simulink model "uas_main_ros2"  (R2026a)
settings: Solver=FixedStepAuto  StopTime=Inf  FixedStep=sample_time
model workspace: external: MAT-File (data not in the file)
values from neighbouring files (symbols this model uses):
  arm_length = 0.17    [uas_parameters.m]
  axes_msg = zeros(1, 124)    [uas_parameters.m]
  button_msg = zeros(1, 124)    [uas_parameters.m]
  drag_coefficient = 0.47    [uas_parameters.m]
  g = 9.81    [PosControllerSystem.m]    (also in uas_parameters.m = 9.80665)
  inertia_xx = 0.007    [uas_parameters.m]
  inertia_yy = 0.007    [uas_parameters.m]
  inertia_zz = 0.012    [uas_parameters.m]
  mass_drone = 0.04    [uas_parameters.m]
  mass_total = 0.04    [PosControllerSystem.m]    (also in uas_parameters.m)
  max_rot_velocity = 838    [uas_parameters.m]
  mix_matrix = inv(motor_constant * allocation_matrix)    [uas_parameters.m]
  moment_constant = 0.016    [uas_parameters.m]
  motor_constant = 8.54858e-06    [uas_parameters.m]
  N = size(waypoints, 1)    [quintic_interp.m]
  reference_area = pi * 75e-3^2    (= 0.0176714586764)    [uas_parameters.m]
  rotor_offset_top = 0.01    [uas_parameters.m]
  route = [0 0 1 ; 9 0 1 ; 9 9 1]    [uas_parameters.m]
  sample_time = 4e-2    (= 0.04)    [uas_parameters.m]
  x0 = 36    [uas_parameters.m]
  y0 = 80    [uas_parameters.m]
  z0 = 1    [uas_parameters.m]
undefined symbols (not defined in the file or in its folder): axes, axes_SL_Info, buttons, buttons_SL_Info, poly_traj, quat2rotm, X, Y, Z
libraries: nesl_utility x32, sm_lib x25, ros2lib x16, dspfdesign x3, simulink x2, sharedtransform x2, sim3dlib x1, uavsim3dlib x1, vrlib x1
(part 1 of 3)
settings Model: Creator=david  LastModifiedBy=mello
settings OptimizationCC: PassReuseOutputArgsThreshold=0.0
settings DebuggingCC: UnderSpecifiedDimensionMsg=warning
settings HardwareCC: ProdHWDeviceType=Generic->Unspecified (assume 32-bit Generic)  UseEmbeddedCoderFeatures=off
settings SFSimCC: SimTargetLang=C++
settings RTWCC: SystemTargetFile=ert.tlc  HardwareBoard=Robot Operating System (ROS)  TLCOptions="-aInlineSetEventsForThisBaseRateFcn=TLC_FALSE -aSuppressMultiTaskScheduler=TLC_FALSE  -aRateBasedStepFcn=0"  Toolchain=Catkin  TargetLang=C++  Description=Embedded Coder
settings ERTTargetCC: RootIOFormat=Structure reference  DynamicArrayContainerType=coder::array  ERTCustomFileBanners=off  CodeInterfacePackaging=C++ class  SupportContinuousTime=on  SupportNonInlinedSFcns=on  ModelStepFunctionPrototypeControlCompliant=off
settings SimscapeCC: SimscapeNominalValues="[{\"value\":\"1\",\"unit\":\"A\"},{\"value\":\"1\",\"unit\":\"bar\"},{\"value\":\"1\",\"unit\":\"cm^2\"},{\"value\":\"1\",\"unit\":\"cm^3/s\"},{\"value\":\"1\",\"unit\":\"kJ/kg\"},{\"value\":\"1\",\"unit\":\"kW\"},{\"value\":\"1\",\"unit\":\"l\"},{\"value\":\"1\",\"unit\":\"N\"},{\"value\":\"1\",\"unit\":\"N*m\"},{\"value\":\"1\",\"unit\":\"V\"}]"  SimscapeLogSimulationStatistics=on
settings ExplorerConfigSet: InternalSimMechanicsExplorerSettings="<ExplorerConfiguration><canonicalview>default</canonicalview><AnimationSetting><BasePlaybackSpeed>1.0</BasePlaybackSpeed><PlaybackSpeedFactor>1.0</PlaybackSpeedFactor></AnimationSetting><TilePanel><TileInfo><Tiles Columns=\"1\" Count=\"1\" Rows=\"1\"><Column Weight=\"1\"/><Row Weight=\"1\"/><Tile Height=\"1\" Width=\"1\" X=\"0\" Y=\"0\"/></Tiles></TileInfo><SceneInfo><SceneViewer><BGColor><R>0.400000005960464478</R><G>0.400000005960464478</G><B>0.400000005960464478</B></BGColor><Camera><DoPerspective>off</DoPerspective><Position><X>7.41918867546502359</X><Y>0.562842449888731333</Y><Z>8.36768126399918444</Z></Position><Center><X>4.24878770726833288</X><Y>4.27540210027623324</Y><Z>0.996100590645515815</Z></Center><Up><X>-0.578313069199200891</X><Y>0.601173295476169489</Y><Z>0.551493121262380703</Z></Up><ViewLimDist>1</ViewLimDist><YLim>5.48746925830841104</YLim><XLim>8.41878250057976274</XLim></Camera></SceneViewer></SceneInfo></TilePanel><MechEditorPanel><Cameras/><GfxPanelCameraMap/><VideoCreator><PlaybackSpeedRatio>1.0</PlaybackSpeedRatio><FrameRate>30</FrameRate><VideoFormat>Motion JPEG AVI</VideoFormat><FrameSize>auto</FrameSize></VideoCreator></MechEditorPanel></ExplorerConfiguration>"

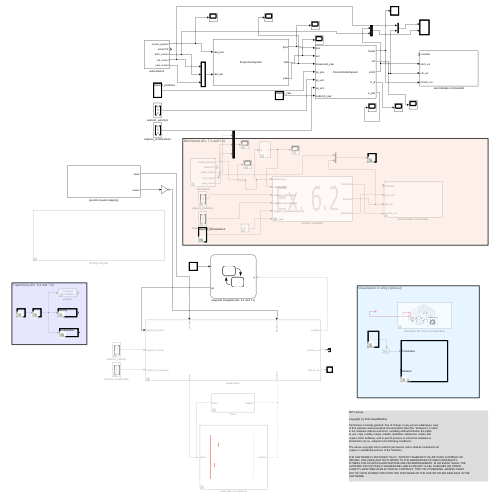
[thumbnail: Simulink's stored preview of the top-level diagram]
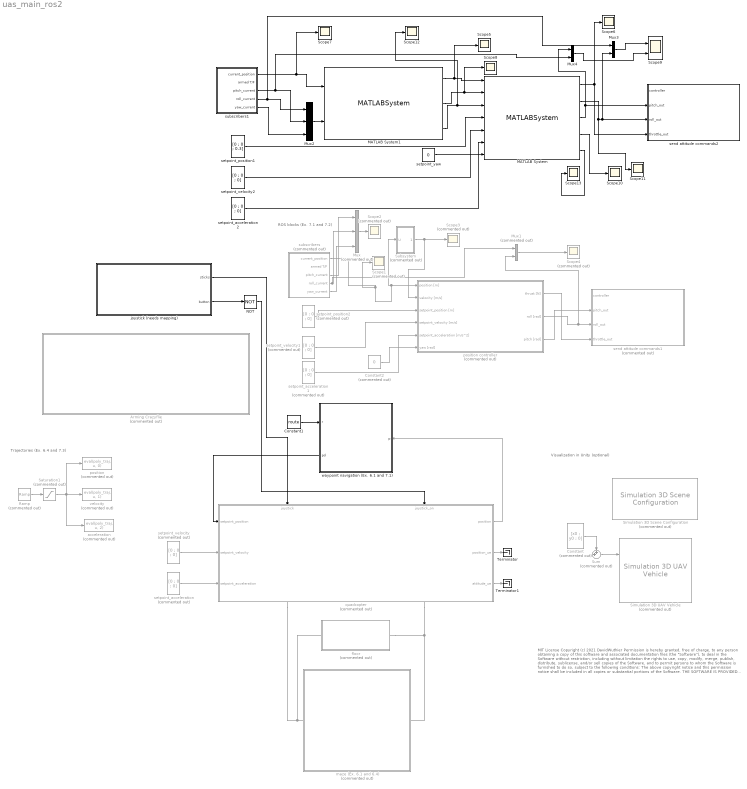
== system uas_main_ros2 ==
  note: MIT License
      |
      | Copyright (c) 2021 DavidWuthier
      |
      | Permission is hereby granted, free of charge, to any person obtaining a copy
      | of this software and associated documentation files (the "Software"), to deal
      | in the Software without restriction, including without limitation the rights
      | to use, copy, modify, merge, publish, distribute, sublicense, and/or sell
      | copies of the Software, and to permit persons to whom the Software is
      | furnished to do so, subject to the following conditions:
      |
      | The above copyright notice and this permission notice shall be included in all
      | copies or substantial portions of the Software.
      |
      | THE SOFTWARE IS PROVIDED "AS IS", WITHOUT WARRANTY OF ANY KIND, EXPRESS OR
      | IMPLIED, INCLUDING BUT NOT LIMITED TO THE WARRANTIES OF MERCHANTABILITY,
      | FITNESS FOR A PARTICULAR PURPOSE AND NONINFRINGEMENT. IN NO EVENT SHALL THE
      | AUTHORS OR COPYRIGHT HOLDERS BE LIABLE FOR ANY CLAIM, DAMAGES OR OTHER
      | LIABILITY, WHETHER IN AN ACTION OF CONTRACT, TORT OR OTHERWISE, ARISING FROM,
      | OUT OF OR IN CONNECTION WITH THE SOFTWARE OR THE USE OR OTHER DEALINGS IN THE
      | SOFTWARE.
  note: Visualization in Unity (optional)
  note: Trajectories (Ex. 6.4 and 7.3)
  note: ROS blocks (Ex. 7.1 and 7.2)
  Arming Crazyflie : Subsystem  Commented=on
  Constant : Constant  Commented=on  Value=[x0 ; y0 ; 0]  VectorParams1D=off
  Constant1 : Constant  Value=route
  Constant2 : Constant  Commented=on  Value=0
  MATLAB System : MATLABSystem  System=PosControllerSystem  SimulateUsing=Code generation
      mask Type: PosControllerSystem
  MATLAB System1 : MATLABSystem  System=PreprocessSystem  SimulateUsing=Interpreted execution
      mask Type: PreprocessSystem
  Mux : Mux  Commented=on  Inputs=3
  Mux1 : Mux  Commented=on  Inputs=2
  Mux2 : Mux  Inputs=3
  Mux3 : Mux  Inputs=2
  Mux4 : Mux  Inputs=2
  NOT : Logic  Operator=NOT  IconShape=distinctive  AllPortsSameDT=off  OutDataTypeStr=boolean
  Ramp : simulink/Sources/Ramp  Commented=on  slope=1  start=0  InitialOutput=0
  Saturation1 : Saturate  Commented=on  UpperLimit=knots(end)  LowerLimit=0
  Scope{1..4} (4 alike) : Scope  Commented=on
      Scope1 settings: ActiveDisplayYMinimum=-3.62331068311887  ActiveDisplayYMaximum=5.4527683046975284  DataLoggingVariableName=ScopeData2
      Scope2 settings: ActiveDisplayYMinimum=-3.9205477094873689  ActiveDisplayYMaximum=3.9221624092985992  DataLoggingVariableName=ScopeData8
      Scope3 settings: ActiveDisplayYMinimum=-0.704351972070756  ActiveDisplayYMaximum=1.1465122899088067
      Scope4 settings: ActiveDisplayYMinimum=-2.2453805222482135  ActiveDisplayYMaximum=0.97073912636413651  DataLoggingVariableName=ScopeData9
  Scope{5..8,10..13} (8 alike) : Scope
      Scope10 settings: ActiveDisplayYMinimum=-0.2913419984889255  ActiveDisplayYMaximum=0.16018686807512672  DataLoggingVariableName=ScopeData16
      Scope11 settings: ActiveDisplayYMinimum=-7.8906329945921971  ActiveDisplayYMaximum=8.2581334209704433  DataLoggingVariableName=ScopeData17
      Scope12 settings: ActiveDisplayYMinimum=-3.5797770650115455  ActiveDisplayYMaximum=6.1446597978088091  DataLoggingVariableName=ScopeData18
      Scope13 settings: ActiveDisplayYMinimum=-2.1801041636378873  ActiveDisplayYMaximum=1.2366941298563761  DataLoggingVariableName=ScopeData19
      Scope5 settings: ActiveDisplayYMinimum=-1.3039902181688128  ActiveDisplayYMaximum=1.1270222818311879  DataLoggingVariableName=ScopeData10
      Scope6 settings: ActiveDisplayYMinimum=-0.96457637394383644  ActiveDisplayYMaximum=1.4435775810644444  DataLoggingVariableName=ScopeData11
      Scope7 settings: ActiveDisplayYMinimum=-18.731354302133511  ActiveDisplayYMaximum=13.426335857782668  DataLoggingVariableName=ScopeData12
      Scope8 settings: ActiveDisplayYMinimum=-3.9205477094873689  ActiveDisplayYMaximum=3.9221624092985992  DataLoggingVariableName=ScopeData13
  Scope9 : Scope  NumInputPorts=2
      settings: ActiveDisplayYMinimum=-11.154686865264761  ActiveDisplayYMaximum=4.93616611048231  DataLoggingVariableName=ScopeData15
  Simulation 3D Scene Configuration : sim3dlib/Simulation 3D Scene Configuration  Priority=0  Commented=on  ProjectFormat=Default Scenes  SceneDesc=US city block  ProjectName=/usr/local/MATLAB/R2026a/toolbox/shared/sim3d_projects/automotive_project_linux/UE/LinuxNoEditor/VehicleSimulation.sh  ScenePath=/Game/Maps/USCityBlock  EnableOpenDRIVE=off  vehTagList={'Scene Origin';'SimulinkVehicle1'}  vehTag=SimulinkVehicle1  AttachedCameraRelativeTranslation=[0 0 0]  FreeCameraDefaultInitialTranslation=[-6, 0, 2]  AttachedCameraRelativeRotation=[0 0 0]  FreeCameraDefaultInitialRotation=[0, -15, 0]  ViewpointName=Custom  FreeCameraInitialTranslation=[0, 0, 0]  FreeCameraInitialRotation=[0, 0, 0]  OpVisEn=off  Ts=sample_time  EnableWindow=on  EnableRemoteAccess=off  SimulationMode=CoSimulation  SimulateUsing=Interpreted execution  EnableAnimationRecording=off  OverrideDefaultRecording=off  AnimationRecordingFileName=sim3dAnimation.mat  AnimationRecordingInterval=[0 inf]  EnableWeather=off  SunAzimuth=90  SunAltitude=40.0  EnableGeospatialSun=off  Latitude=0  Longitude=0  Date=2023-01-01  Time=10:30:00  GeoTimeZone=-5.0  SunDaylightSaving=off  wind=1  clouds=10  EnableVolumetricClouds=off  CloudCoverage=0  CloudAltitude=6  fog=0  rain=0  RaindropsEffect=off  SnowDensity=0  EnableGeospatial=off  TilesetSource=Earth terrain  UseTrueOrigin=off  OriginHeight=200  OriginLatitude=40.744652  OriginLongitude=-73.988864  MapStyle=Aerial  AdditionalAssetIDs=[]  UseAdvancedSunSky=off  SolarTime=11  TimeZone=-5  Day=21  Month=9  Year=2022  UseDaylightSavingTime=on  DSTStartDay=10  DSTStartMonth=3  DSTEndDay=3  DSTEndMonth=11  DSTSwitchHour=2  sensorTag=MainCamera1  sensorId=1  sensorName=MainCamera1  mountLoc=Origin  offsetFlag=off  tmountOffset=[0, 0, 0]  rmountOffset=[0, 0, 0]  HorizontalResolution=1280  VerticalResolution=720  HorizontalFOV=60  mountPoint=[0 0 0]  mountOrientation=[0 0 0]  aMode=4  ID=1  GeoTrigger=Inactive  ViewNameList={'Custom'}  ViewTranslationList={'[0 0 0]'}  ViewRotationList={'[0 0 0]'}
      settings: LibrarySourceBlock=uavsim3dlib/Simulation 3D Scene Configuration
  Simulation 3D UAV Vehicle : uavsim3dlib/Simulation 3D UAV Vehicle  Commented=on  Mesh=Quadrotor  MeshPath=/MathWorksUAVContent/UAVs/HexaRotorUAV/HexaRotor.HexaRotor  Color=Black  ActorName=SimulinkVehicle1  UseGlobalFrame=off  InitialTranslation=[x0 y0 z0]  InitialRotation=[0 0 0]  InitialTranslationGlobal=[0 0 0]  InitialGeoOrigin=[0 0 0]  InitialRotationGlobal=[0 0 0]  SampleTime=-1  ActorType=SimulinkVehicle  ID=1  aMode=4  ActorTag=SimulinkVehicle1
  Subsystem : Subsystem  Commented=on
  Sum : Sum  Commented=on  Inputs=++|
  Terminator : Terminator
  Terminator1 : Terminator
  acceleration : MATLABFcn  Commented=on  MATLABFcn=eval(poly_traj, u, 2)  OutputDimensions=[3 1]  Output1D=off
  floor : Subsystem  Commented=on
  joystick (needs mapping) : Subsystem
  maze (Ex. 6.1 and 6.4) : Subsystem  Commented=on
      mask Display: image('$imagefile'); % Use "Edit Image" on toolstrip to change.
  position : MATLABFcn  Commented=on  MATLABFcn=eval(poly_traj, u, 0)  OutputDimensions=[3 1]  Output1D=off
  position controller : Subsystem  Commented=on
      mask Display: image('$imagefile'); % Use "Edit Image" on toolstrip to change.
  quadcopter : Subsystem  Commented=on
      settings: PortSchema="{\"entries\":[{\"content\":{\"sides\":[{\"content\":{\"connectorIds\":[\"In1\",\"In2\",\"In3\"]},\"type\":\"ConnectorPlacement.EquallySpacedRectSide\",\"uuid\":\"ed16c4a7-5f5f-48d5-8471-b227eef37b0b\"},{\"content\":{\"connectorIds\":[\"Out1\",\"Out2\",\"Out3\"],\"side\":\"RIGHT\"},\"type\":\"ConnectorPlacement.EquallySpacedRectSide\",\"uuid\":\"303ea24f-0a15-469a-b5d8-cc8b33d29b5f\"},{\"content\":{\"connectorIds\":[\"In4\",\"In5\"],\"side\":\"TOP\"},\"type\":\"ConnectorPlacement.EquallySpacedRectSide\",\"uuid\":\"d3970502-0872-434b-b7c5-387e72ad4178\"},{\"content\":{\"connectorIds\":[\"RConn1\",\"RConn2\"],\"side\":\"BOTTOM\"},\"type\":\"ConnectorPlacement.EquallySpacedRectSide\",\"uuid\":\"dd808c8e-2f91-44fb-8d51-5dec3bd81dd9\"}]},\"type\":\"ConnectorPlacement.EquallySpacedConnector\",\"uuid\":\"aacf4a84-08b7-4fd3-a02a-51c4e2a4df71\"}],\"packageUris\":[\"http://schema.mathworks.com/mf0/Connector/R2020b\"],\"version\":\"1.0\"}"
  send attitude commands1 : Subsystem  Commented=on
  send attitude commands2 : Subsystem
  setpoint_acceleration : Constant  Commented=on  Value=[0 ; 0 ; 0]  VectorParams1D=off
  setpoint_acceleration1 : Constant  Commented=on  Value=[0 ; 0 ; 0]  VectorParams1D=off
  setpoint_acceleration2 : Constant  Value=[0 ; 0 ; 0]  VectorParams1D=off
  setpoint_position1 : Constant  Value=[0 ; 0 ; 0.3]  VectorParams1D=off
  setpoint_position2 : Constant  Commented=on  Value=[0 ; 0 ; 0]  VectorParams1D=off
  setpoint_velocity : Constant  Commented=on  Value=[0 ; 0 ; 0]  VectorParams1D=off
  setpoint_velocity1 : Constant  Commented=on  Value=[0 ; 0 ; 0]  VectorParams1D=off
  setpoint_velocity2 : Constant  Value=[0 ; 0 ; 0]  VectorParams1D=off
  setpoint_yaw : Constant  Value=0
  subscribers : Subsystem  Commented=on
  subscribers1 : Subsystem
  velocity : MATLABFcn  Commented=on  MATLABFcn=eval(poly_traj, u, 1)  OutputDimensions=[3 1]  Output1D=off
  waypoint navigation (Ex. 6.1 and 7.1) : Stateflow chart  TreatAsAtomicUnit=on
      settings: PortSchema="{\"entries\":[{\"content\":{\"sides\":[{\"content\":{\"connectorIds\":[\"In1\",\"Out1\"]},\"type\":\"ConnectorPlacement.EquallySpacedRectSide\",\"uuid\":\"7c2fff0d-1179-4786-9432-1971d7acd904\"},{\"content\":{\"connectorIds\":[\"In2\"],\"side\":\"RIGHT\"},\"type\":\"ConnectorPlacement.EquallySpacedRectSide\",\"uuid\":\"377a8206-b310-41c0-9a17-faf5318c89cb\"},{\"content\":{\"connectorIds\":[],\"side\":\"TOP\"},\"type\":\"ConnectorPlacement.EquallySpacedRectSide\",\"uuid\":\"b953090a-ffdb-4e30-a5fe-7bef9655f1cf\"},{\"content\":{\"connectorIds\":[],\"side\":\"BOTTOM\"},\"type\":\"ConnectorPlacement.EquallySpacedRectSide\",\"uuid\":\"03dc7a24-529e-4020-b953-d1c4751c5c80\"}]},\"type\":\"ConnectorPlacement.EquallySpacedConnector\",\"uuid\":\"03bac9f4-6480-492d-9af3-57aec4db8fd8\"}],\"packageUris\":[\"http://schema.mathworks.com/mf0/Connector/R2020b\"],\"version\":\"1.0\"}"
  wires:
  Sum/1 -> Simulation 3D UAV Vehicle/1
  Constant/1 -> Sum/1
  Constant1/1 -> waypoint navigation (Ex. 6.1 and 7.1)/1(r)
  Saturation1/1 -> acceleration/1, position/1, velocity/1
  Ramp/1 -> Saturation1/1
  setpoint_velocity/1 -> quadcopter/2(setpoint_velocity)
  setpoint_acceleration/1 -> quadcopter/3(setpoint_acceleration)
  NOT/1 -> quadcopter/5(joystick_on)
  joystick (needs mapping)/1(sticks) -> quadcopter/4(joystick)
  joystick (needs mapping)/2(button) -> NOT/1
  quadcopter/1(position) -> waypoint navigation (Ex. 6.1 and 7.1)/2(p)
  waypoint navigation (Ex. 6.1 and 7.1)/1(pd) -> quadcopter/1(setpoint_position)
  quadcopter/2(position_ue) -> Terminator/1
  quadcopter/3(attitude_ue) -> Terminator1/1
  subscribers/1(current_position) -> Subsystem/1(U), position controller/1(position [m]), Scope1/1
  position controller/2(roll [rad]) -> Mux1/2, send attitude commands1/3(roll_out)
  position controller/3(pitch [rad]) -> send attitude commands1/2(pitch_out)
  position controller/1(thrust [N]) -> send attitude commands1/4(throttle_out)
  setpoint_velocity1/1 -> position controller/4(setpoint_velocity [m/s])
  setpoint_acceleration1/1 -> position controller/5(setpoint_acceleration [m/s^2])
  Constant2/1 -> position controller/6(yaw [rad])
  Subsystem/1(Out1) -> position controller/2(velocity [m/s]), Scope3/1
  setpoint_position2/1 -> position controller/3(setpoint_position [m])
  subscribers/3(pitch_current) -> Mux/1
  subscribers/4(roll_current) -> Mux1/1, Mux/2
  subscribers/5(yaw_current) -> Mux/3
  Mux/1 -> Scope2/1
  Mux1/1 -> Scope4/1
  ? -> ?
  MATLAB System1/1 -> MATLAB System/1, Scope5/1
  MATLAB System1/2 -> Scope8/1, MATLAB System/2
  subscribers1/1(current_position) -> Scope7/1, MATLAB System1/1
  subscribers1/4(roll_current) -> Mux3/1, Mux2/1
  subscribers1/3(pitch_current) -> Mux4/2, Mux2/2
  subscribers1/5(yaw_current) -> Mux2/3
  Mux2/1 -> MATLAB System1/2
  MATLAB System/1 -> send attitude commands2/4(throttle_out), Scope6/1
  MATLAB System/2 -> Scope11/1, Mux3/2, send attitude commands2/3(roll_out)
  MATLAB System/3 -> send attitude commands2/2(pitch_out), Mux4/1
  MATLAB System1/3 -> MATLAB System/3, Scope12/1
  setpoint_position1/1 -> MATLAB System/4
  setpoint_velocity2/1 -> MATLAB System/5
  setpoint_acceleration2/1 -> MATLAB System/6
  setpoint_yaw/1 -> MATLAB System/7
  Mux3/1 -> Scope9/1
  Mux4/1 -> Scope9/2
  MATLAB System/4 -> Scope10/1
  MATLAB System/5 -> Scope13/1
  connections:
  floor/LConn1 -- quadcopter/RConn1 -- maze (Ex. 6.1 and 6.4)/LConn1
  floor/RConn1 -- quadcopter/RConn2 -- maze (Ex. 6.1 and 6.4)/RConn1

== system uas_main_ros2/Arming Crazyflie ==
  Arm : Constant  OutDataTypeStr=boolean
  Blank Message : ros2lib/Blank Message  messageClass=Service Request  entityType=crazyflie_interfaces/Arm  messageType=crazyflie_interfaces/ArmRequest  SampleTime=inf
  Bus Assignment : BusAssignment  AssignedSignals=arm
  Call Service : ros2lib/Call Service  topicSource=Specify your own  service=/cf231/arm  serviceType=crazyflie_interfaces/Arm  connectionTimeout=5  ShowErrorCodeOutput=on  legacyBusStruct=off  QOSHistory=Keep last  QOSDepth=1  QOSReliability=Reliable  QOSDurability=Volatile  QOSDeadline=Inf  QOSLifespan=Inf  QOSLiveliness=Automatic  QOSLeaseDuration=Inf  QOSAvoidROSNamespaceConventions=off
  Manual Switch : ManualSwitch
  Terminator2 : Terminator
  Terminator3 : Terminator
  UnArm : Constant  Value=0  OutDataTypeStr=boolean
  wires:
  Blank Message/1 -> Bus Assignment/1
  UnArm/1 -> Manual Switch/1
  Arm/1 -> Manual Switch/2
  Call Service/1 -> Terminator2/1
  Bus Assignment/1 -> Call Service/1
  Manual Switch/1 -> Bus Assignment/2
  Call Service/2 -> Terminator3/1

== system uas_main_ros2/Subsystem ==
  U : Inport
  Demux : Demux  Outputs=3
  Discrete Derivative : simulink/Discrete/Discrete Derivative  gainval=1.0  ICPrevScaledInput=0.0  OutMin=[]  OutMax=[]  OutDataType=fixdt(1, 16)  OutScaling=2^-10  DoSatur=off
  Lowpass Filter : dspfdesign/Lowpass Filter  FilterType=FIR  DesignForMinimumOrder=on  FilterOrder=50  PassbandFrequency=10  StopbandFrequency=25  PassbandRipple=5  StopbandAttenuation=80  SampleRateMode=Specify on dialog  SampleRate=100  SimulateUsing=Interpreted execution  roundingMode=Floor  coeffsDataTypeStr=fixdt(1,16)
  Lowpass Filter1 : dspfdesign/Lowpass Filter  FilterType=FIR  DesignForMinimumOrder=on  FilterOrder=50  PassbandFrequency=10  StopbandFrequency=25  PassbandRipple=5  StopbandAttenuation=80  SampleRateMode=Specify on dialog  SampleRate=100  SimulateUsing=Interpreted execution  roundingMode=Floor  coeffsDataTypeStr=fixdt(1,16)
  Lowpass Filter2 : dspfdesign/Lowpass Filter  FilterType=FIR  DesignForMinimumOrder=on  FilterOrder=50  PassbandFrequency=10  StopbandFrequency=25  PassbandRipple=5  StopbandAttenuation=80  SampleRateMode=Specify on dialog  SampleRate=100  SimulateUsing=Interpreted execution  roundingMode=Floor  coeffsDataTypeStr=fixdt(1,16)
  Mux : Mux  Inputs=3
  Scope2 : Scope
      settings: ActiveDisplayYMinimum=-95.981515086180551  ActiveDisplayYMaximum=68.775458951264923  DataLoggingVariableName=ScopeData3
  Out1 : Outport
  wires:
  Demux/2 -> Lowpass Filter1/1
  Lowpass Filter2/1 -> Mux/3
  Demux/3 -> Lowpass Filter2/1
  Discrete Derivative/1 -> Scope2/1, Demux/1
  Lowpass Filter1/1 -> Mux/2
  Demux/1 -> Lowpass Filter/1
  Lowpass Filter/1 -> Mux/1
  Mux/1 -> Out1/1
  U/1 -> Discrete Derivative/1

== system uas_main_ros2/floor ==
  Brick Solid1 : sm_lib/Body Elements/Brick Solid  BrickDimensions=[3 3 0.1]  BrickDimensionsUnits=m  ExportEntireGeometry=on  InertiaType=CalculateFromGeometry  BasedOnType=Density  Density=0  DensityUnits=kg/m^3  Mass=1  MassUnits=kg  CenterOfMass=[0 0 0]  CenterOfMassUnits=m  MomentsOfInertia=[1 1 1]  MomentsOfInertiaUnits=kg*m^2  ProductsOfInertia=[0 0 0]  ProductsOfInertiaUnits=kg*m^2  GraphicType=FromGeometry  MarkerShape=Sphere  MarkerSize=10  GraphicVisPropType=SimpleVisualProperties  GraphicDiffuseColor=[0.4 0.4 0.4]  GraphicOpacity=1  GraphicSpecularColor=[0.5 0.5 0.5 1.0]  GraphicAmbientColor=[0.15 0.15 0.15 1.0]  GraphicEmissiveColor=[0.0 0.0 0.0 1.0]  GraphicShininess=75  DoExposeReferenceFrame=on  SerializedFrames=<Frames/>
  Rigid Transform5 : sm_lib/Frames and Transforms/Rigid Transform  RotationMethod=None  FollAlignAxisA=+X  BaseAlignAxisA=+Y  FollAlignAxisB=+Y  BaseAlignAxisB=+Z  RotationStandardAxis=+Z  RotationAngle=0.0  RotationAngleUnits=deg  RotationArbitraryAxis=[0 0 1]  RotationSequenceAxes=FollowerAxes  RotationSequence=XYX  RotationSequenceAngles=[0 0 0]  RotationSequenceAnglesUnits=deg  RotationMatrix=[1 0 0; 0 1 0; 0 0 1]  Quaternion=[1 0 0 0]  TranslationMethod=StandardAxis  TranslationCartesianOffset=[0 0 0]  TranslationCartesianOffsetUnits=m  TranslationStandardAxis=-Z  TranslationStandardOffset=0.05  TranslationStandardOffsetUnits=m  TranslationROffset=0  TranslationROffsetUnits=m  TranslationThetaOffset=0  TranslationThetaOffsetUnits=deg  TranslationZOffset=0  TranslationZOffsetUnits=m
  Spatial Contact Force : sm_lib/Forces and Torques/Spatial Contact Force  SenseSeparationDistance=off  NormalForceType=SmoothSpringDamper  NormalStiffness=stiffness_wall  NormalStiffnessUnits=N/m  NormalDamping=critical_damping_wall  NormalDampingUnits=N/(m/s)  NormalTransitionRegionWidth=1e-4  NormalTransitionRegionWidthUnits=m  FrictionType=SmoothStickSlip  CoefficientOfStaticFriction=0.5  CoefficientOfDynamicFriction=0.3  FrictionalCriticalVelocity=1e-3  FrictionalCriticalVelocityUnits=m/s  SenseContactSignal=off  SensePenetrationDepth=off  SenseNormalVelocity=off  SenseTangentialVelocity=off  SensingForceTorqueDirection=BaseOnFollower  SensingForceTorqueResolutionFrame=ContactFrame  SenseNormalForce=off  SenseNormalForceMagnitude=off  SenseNormalTorque=off  SenseFrictionalForce=off  SenseFrictionalForceMagnitude=off  SenseFrictionalTorque=off  SenseTotalForce=off  SenseTotalTorque=off  SenseContactBaseRotation=off  SenseContactBaseTranslation=off  SenseContactFollowerRotation=off  SenseContactFollowerTranslation=off  ZeroCrossDetectContactStartAndEnd=off
  base : PMIOPort  Side=Left
  collision : PMIOPort  Port=2  Side=Right
  connections:
  Rigid Transform5/RConn1 -- Brick Solid1/RConn1
  Rigid Transform5/LConn1 -- base/RConn1
  Spatial Contact Force/RConn1 -- Brick Solid1/LConn1
  Spatial Contact Force/LConn1 -- collision/RConn1

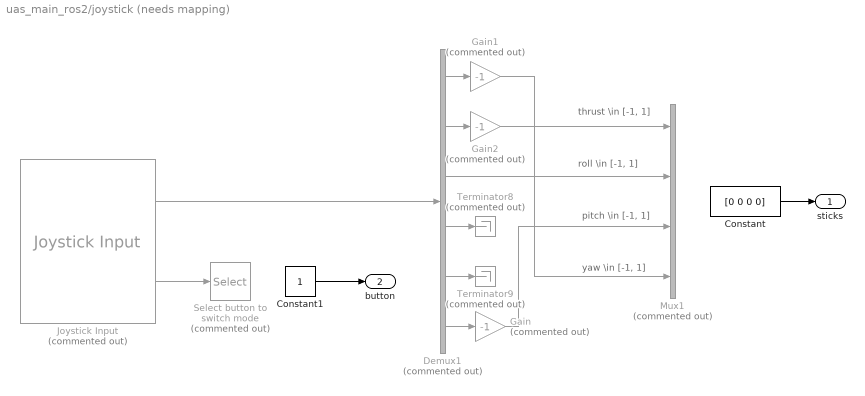
== system uas_main_ros2/joystick (needs mapping) ==
  note: thrust \in [-1, 1]
  note: roll \in [-1, 1]
  note: pitch \in [-1, 1]
  note: yaw \in [-1, 1]
  Constant : Constant  Value=[0 0 0 0]
  Constant1 : Constant
  Demux1 : Demux  Commented=on  Outputs=6
  Gain : Gain  Commented=on  Gain=-1
  Gain1 : Gain  Commented=on  Gain=-1
  Gain2 : Gain  Commented=on  Gain=-1
  Joystick Input : vrlib/Joystick Input  Commented=on  joyid=1  adjustports=on  forcefeed=off
  Mux1 : Mux  Commented=on
  Select button to switch mode : Selector  Commented=on  InputPortWidth=15  IndexOptions=Index vector (dialog)  Indices=8  OutputSizes=1
  Terminator8 : Terminator  Commented=on
  Terminator9 : Terminator  Commented=on
  sticks : Outport
  button : Outport  Port=2
  wires:
  Gain1/1 -> Mux1/4
  Joystick Input/1 -> Demux1/1
  Gain2/1 -> Mux1/1
  Demux1/1 -> Gain1/1
  Joystick Input/2 -> Select button to switch mode/1
  Demux1/6 -> Gain/1
  Demux1/5 -> Terminator9/1
  Demux1/3 -> Mux1/2
  Demux1/2 -> Gain2/1
  Demux1/4 -> Terminator8/1
  Gain/1 -> Mux1/3
  Constant/1 -> sticks/1
  Constant1/1 -> button/1

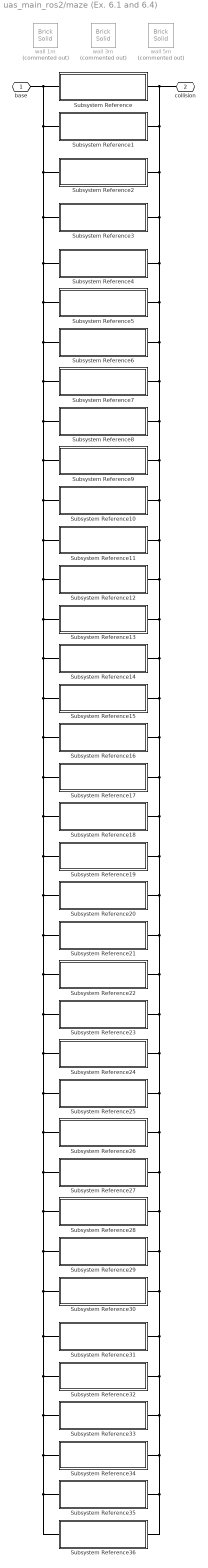
== system uas_main_ros2/maze (Ex. 6.1 and 6.4) ==
  Subsystem Reference : Subsystem  ReferencedSubsystem=uas_wall  l=5  x=-1  y=1.5  yaw=0
  Subsystem Reference1 : Subsystem  ReferencedSubsystem=uas_wall  l=5  x=-1  y=7.5  yaw=0
  Subsystem Reference10 : Subsystem  ReferencedSubsystem=uas_wall  l=5  x=7.5  y=10  yaw=pi/2
  Subsystem Reference11 : Subsystem  ReferencedSubsystem=uas_wall  l=5  x=5  y=10  yaw=pi/2
  Subsystem Reference12 : Subsystem  ReferencedSubsystem=uas_wall  l=5  x=1.5  y=1  yaw=pi/2
  Subsystem Reference13 : Subsystem  ReferencedSubsystem=uas_wall  l=3  x=4.5  y=1  yaw=pi/2
  Subsystem Reference14 : Subsystem  ReferencedSubsystem=uas_wall  l=3  x=8  y=2.5  yaw=0
  Subsystem Reference15 : Subsystem  ReferencedSubsystem=uas_wall  l=1  x=6  y=4.5  yaw=0
  Subsystem Reference16 : Subsystem  ReferencedSubsystem=uas_wall  l=1  x=6  y=1.5  yaw=0
  Subsystem Reference17 : Subsystem  ReferencedSubsystem=uas_wall  l=1  x=2  y=1.5  yaw=0
  Subsystem Reference18 : Subsystem  ReferencedSubsystem=uas_wall  l=1  x=0  y=2.5  yaw=0
  Subsystem Reference19 : Subsystem  ReferencedSubsystem=uas_wall  l=5  x=5.5  y=4  yaw=pi/2
  Subsystem Reference2 : Subsystem  ReferencedSubsystem=uas_wall  l=5  x=-1  y=5  yaw=0
  Subsystem Reference20 : Subsystem  ReferencedSubsystem=uas_wall  l=1  x=4  y=3.5  yaw=0
  Subsystem Reference21 : Subsystem  ReferencedSubsystem=uas_wall  l=1  x=2.5  y=4  yaw=pi/2
  Subsystem Reference22 : Subsystem  ReferencedSubsystem=uas_wall  l=1  x=0.5  y=2  yaw=pi/2
  Subsystem Reference23 : Subsystem  ReferencedSubsystem=uas_wall  l=1  x=1.5  y=2  yaw=pi/2
  Subsystem Reference24 : Subsystem  ReferencedSubsystem=uas_wall  l=1  x=-0.5  y=3  yaw=pi/2
  Subsystem Reference25 : Subsystem  ReferencedSubsystem=uas_wall  l=1  x=2  y=4.5  yaw=0
  Subsystem Reference26 : Subsystem  ReferencedSubsystem=uas_wall  l=1  x=1.5  y=5  yaw=pi/2
  Subsystem Reference27 : Subsystem  ReferencedSubsystem=uas_wall  l=1  x=0.5  y=7  yaw=pi/2
  Subsystem Reference28 : Subsystem  ReferencedSubsystem=uas_wall  l=1  x=1  y=7.5  yaw=0
  Subsystem Reference29 : Subsystem  ReferencedSubsystem=uas_wall  l=2  x=8  y=7  yaw=0
  Subsystem Reference3 : Subsystem  ReferencedSubsystem=uas_wall  l=5  x=10  y=1.5  yaw=0
  Subsystem Reference30 : Subsystem  ReferencedSubsystem=uas_wall  l=1  x=-0.5  y=7  yaw=pi/2
  Subsystem Reference31 : Subsystem  ReferencedSubsystem=uas_wall  l=1  x=6  y=5.5  yaw=0
  Subsystem Reference32 : Subsystem  ReferencedSubsystem=uas_wall  l=5  x=5.5  y=8  yaw=pi/2
  Subsystem Reference33 : Subsystem  ReferencedSubsystem=uas_wall  l=1  x=3.5  y=7  yaw=pi/2
  Subsystem Reference34 : Subsystem  ReferencedSubsystem=uas_wall  l=1  x=3  y=7.5  yaw=0
  Subsystem Reference35 : Subsystem  ReferencedSubsystem=uas_wall  l=1  x=4  y=6.5  yaw=0
  Subsystem Reference36 : Subsystem  ReferencedSubsystem=uas_wall  l=1  x=4  y=7.5  yaw=0
  Subsystem Reference4 : Subsystem  ReferencedSubsystem=uas_wall  l=5  x=10  y=7.5  yaw=0
  Subsystem Reference5 : Subsystem  ReferencedSubsystem=uas_wall  l=5  x=10  y=5  yaw=0
  Subsystem Reference6 : Subsystem  ReferencedSubsystem=uas_wall  l=5  x=1.5  y=-1  yaw=pi/2
  Subsystem Reference7 : Subsystem  ReferencedSubsystem=uas_wall  l=5  x=7.5  y=-1  yaw=pi/2
  Subsystem Reference8 : Subsystem  ReferencedSubsystem=uas_wall  l=5  x=5  y=-1  yaw=pi/2
  Subsystem Reference9 : Subsystem  ReferencedSubsystem=uas_wall  l=5  x=1.5  y=10  yaw=pi/2
  wall 1m : sm_lib/Body Elements/Brick Solid  Commented=on  BrickDimensions=[0.1 1 2]  BrickDimensionsUnits=m  ExportEntireGeometry=on  InertiaType=CalculateFromGeometry  BasedOnType=Density  Density=1000  DensityUnits=kg/m^3  Mass=1  MassUnits=kg  CenterOfMass=[0 0 0]  CenterOfMassUnits=m  MomentsOfInertia=[1 1 1]  MomentsOfInertiaUnits=kg*m^2  ProductsOfInertia=[0 0 0]  ProductsOfInertiaUnits=kg*m^2  GraphicType=FromGeometry  MarkerShape=Sphere  MarkerSize=10  GraphicVisPropType=SimpleVisualProperties  GraphicDiffuseColor=wall_color  GraphicOpacity=1.0  GraphicSpecularColor=[0.5 0.5 0.5 1.0]  GraphicAmbientColor=[0.15 0.15 0.15 1.0]  GraphicEmissiveColor=[0.0 0.0 0.0 1.0]  GraphicShininess=75  DoExposeReferenceFrame=on  SerializedFrames=<Frames/>
  wall 3m : sm_lib/Body Elements/Brick Solid  Commented=on  BrickDimensions=[0.1 3 2]  BrickDimensionsUnits=m  ExportEntireGeometry=on  InertiaType=CalculateFromGeometry  BasedOnType=Density  Density=1000  DensityUnits=kg/m^3  Mass=1  MassUnits=kg  CenterOfMass=[0 0 0]  CenterOfMassUnits=m  MomentsOfInertia=[1 1 1]  MomentsOfInertiaUnits=kg*m^2  ProductsOfInertia=[0 0 0]  ProductsOfInertiaUnits=kg*m^2  GraphicType=FromGeometry  MarkerShape=Sphere  MarkerSize=10  GraphicVisPropType=SimpleVisualProperties  GraphicDiffuseColor=wall_color  GraphicOpacity=1.0  GraphicSpecularColor=[0.5 0.5 0.5 1.0]  GraphicAmbientColor=[0.15 0.15 0.15 1.0]  GraphicEmissiveColor=[0.0 0.0 0.0 1.0]  GraphicShininess=75  DoExposeReferenceFrame=on  SerializedFrames=<Frames/>
  wall 5m : sm_lib/Body Elements/Brick Solid  Commented=on  BrickDimensions=[0.1 5 2]  BrickDimensionsUnits=m  ExportEntireGeometry=on  InertiaType=CalculateFromGeometry  BasedOnType=Density  Density=1000  DensityUnits=kg/m^3  Mass=1  MassUnits=kg  CenterOfMass=[0 0 0]  CenterOfMassUnits=m  MomentsOfInertia=[1 1 1]  MomentsOfInertiaUnits=kg*m^2  ProductsOfInertia=[0 0 0]  ProductsOfInertiaUnits=kg*m^2  GraphicType=FromGeometry  MarkerShape=Sphere  MarkerSize=10  GraphicVisPropType=SimpleVisualProperties  GraphicDiffuseColor=wall_color  GraphicOpacity=1.0  GraphicSpecularColor=[0.5 0.5 0.5 1.0]  GraphicAmbientColor=[0.15 0.15 0.15 1.0]  GraphicEmissiveColor=[0.0 0.0 0.0 1.0]  GraphicShininess=75  DoExposeReferenceFrame=on  SerializedFrames=<Frames/>
  base : PMIOPort  Side=Left
  collision : PMIOPort  Port=2  Side=Right
  connections:
  Subsystem Reference35/LConn1 -- Subsystem Reference36/LConn1 -- base/RConn1 -- Subsystem Reference/LConn1 -- Subsystem Reference1/LConn1 -- Subsystem Reference2/LConn1 -- Subsystem Reference3/LConn1 -- Subsystem Reference4/LConn1 -- Subsystem Reference5/LConn1 -- Subsystem Reference6/LConn1 -- Subsystem Reference7/LConn1 -- Subsystem Reference8/LConn1 -- Subsystem Reference9/LConn1 -- Subsystem Reference10/LConn1 -- Subsystem Reference11/LConn1 -- Subsystem Reference12/LConn1 -- Subsystem Reference13/LConn1 -- Subsystem Reference14/LConn1 -- Subsystem Reference15/LConn1 -- Subsystem Reference16/LConn1 -- Subsystem Reference17/LConn1 -- Subsystem Reference18/LConn1 -- Subsystem Reference19/LConn1 -- Subsystem Reference20/LConn1 -- Subsystem Reference21/LConn1 -- Subsystem Reference22/LConn1 -- Subsystem Reference23/LConn1 -- Subsystem Reference24/LConn1 -- Subsystem Reference25/LConn1 -- Subsystem Reference26/LConn1 -- Subsystem Reference27/LConn1 -- Subsystem Reference28/LConn1 -- Subsystem Reference29/LConn1 -- Subsystem Reference30/LConn1 -- Subsystem Reference31/LConn1 -- Subsystem Reference32/LConn1 -- Subsystem Reference33/LConn1 -- Subsystem Reference34/LConn1
  Subsystem Reference32/RConn1 -- Subsystem Reference36/RConn1 -- Subsystem Reference35/RConn1 -- Subsystem Reference34/RConn1 -- Subsystem Reference33/RConn1 -- collision/RConn1 -- Subsystem Reference/RConn1 -- Subsystem Reference1/RConn1 -- Subsystem Reference2/RConn1 -- Subsystem Reference3/RConn1 -- Subsystem Reference4/RConn1 -- Subsystem Reference5/RConn1 -- Subsystem Reference6/RConn1 -- Subsystem Reference7/RConn1 -- Subsystem Reference8/RConn1 -- Subsystem Reference9/RConn1 -- Subsystem Reference10/RConn1 -- Subsystem Reference11/RConn1 -- Subsystem Reference12/RConn1 -- Subsystem Reference13/RConn1 -- Subsystem Reference14/RConn1 -- Subsystem Reference15/RConn1 -- Subsystem Reference16/RConn1 -- Subsystem Reference17/RConn1 -- Subsystem Reference18/RConn1 -- Subsystem Reference19/RConn1 -- Subsystem Reference20/RConn1 -- Subsystem Reference21/RConn1 -- Subsystem Reference22/RConn1 -- Subsystem Reference23/RConn1 -- Subsystem Reference24/RConn1 -- Subsystem Reference25/RConn1 -- Subsystem Reference26/RConn1 -- Subsystem Reference27/RConn1 -- Subsystem Reference28/RConn1 -- Subsystem Reference29/RConn1 -- Subsystem Reference30/RConn1 -- Subsystem Reference31/RConn1

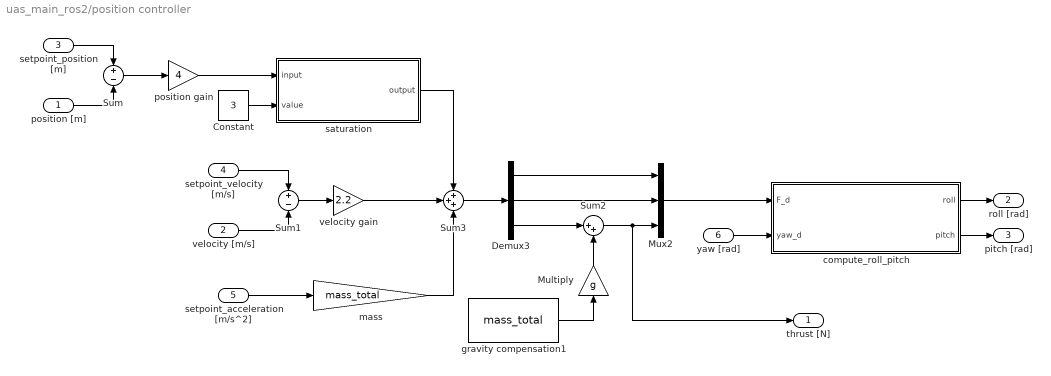
== system uas_main_ros2/position controller ==
  position [m] : Inport
  velocity [m/s] : Inport  Port=2
  setpoint_position [m] : Inport  Port=3
  setpoint_velocity [m/s] : Inport  Port=4
  setpoint_acceleration [m/s^2] : Inport  Port=5
  yaw [rad] : Inport  Port=6
  Constant : Constant  Value=3
  Demux3 : Demux  Outputs=3
  Multiply : Gain  Gain=g
  Mux2 : Mux  Inputs=3
  Sum : Sum  Inputs=+|-
  Sum1 : Sum  Inputs=+|-
  Sum2 : Sum  Inputs=|++
  Sum3 : Sum  Inputs=+++
  compute_roll_pitch : MATLAB Function  TreatAsAtomicUnit=on
  gravity compensation1 : Constant  Value=mass_total  VectorParams1D=off
  mass : Gain  Gain=mass_total
  position gain : Gain  Gain=4
  saturation : Subsystem
  velocity gain : Gain  Gain=2.2
  thrust [N] : Outport
  roll [rad] : Outport  Port=2
  pitch [rad] : Outport  Port=3
  wires:
  saturation/1(output) -> Sum3/1
  position gain/1 -> saturation/1(input)
  gravity compensation1/1 -> Multiply/1
  velocity [m/s]/1 -> Sum1/2
  Demux3/3 -> Sum2/1
  mass/1 -> Sum3/3
  Constant/1 -> saturation/2(value)
  Sum2/1 -> thrust [N]/1, Mux2/3
  Sum1/1 -> velocity gain/1
  velocity gain/1 -> Sum3/2
  Sum/1 -> position gain/1
  Sum3/1 -> Demux3/1
  Demux3/1 -> Mux2/1
  Mux2/1 -> compute_roll_pitch/1(F_d)
  Demux3/2 -> Mux2/2
  compute_roll_pitch/1(roll) -> roll [rad]/1
  Multiply/1 -> Sum2/2
  setpoint_position [m]/1 -> Sum/1
  compute_roll_pitch/2(pitch) -> pitch [rad]/1
  position [m]/1 -> Sum/2
  yaw [rad]/1 -> compute_roll_pitch/2(yaw_d)
  setpoint_velocity [m/s]/1 -> Sum1/1
  setpoint_acceleration [m/s^2]/1 -> mass/1

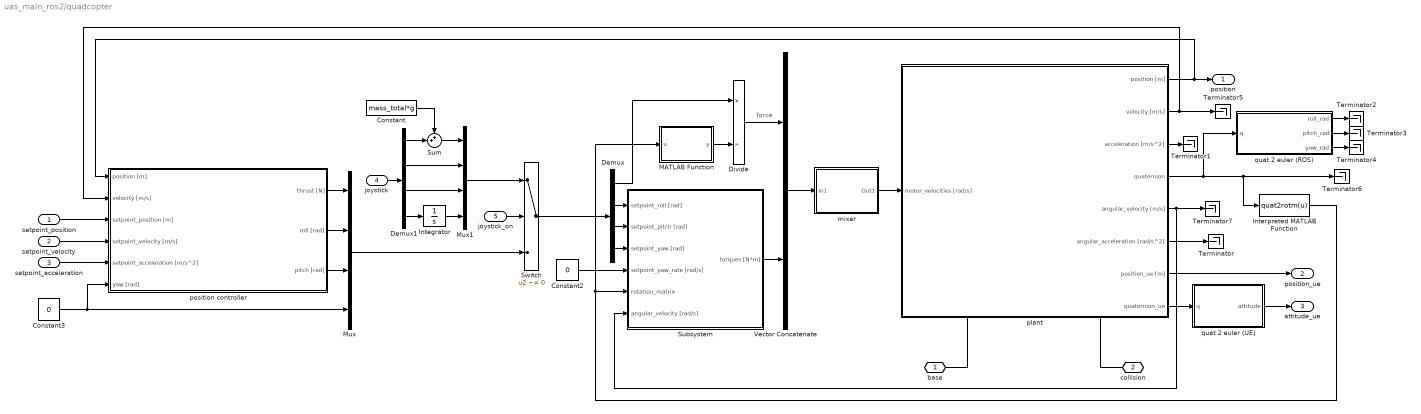
== system uas_main_ros2/quadcopter ==
  note: force
  setpoint_position : Inport
  setpoint_velocity : Inport  Port=2
  setpoint_acceleration : Inport  Port=3
  joystick : Inport  Port=4
  joystick_on : Inport  Port=5
  Constant : Constant  Value=mass_total*g
  Constant2 : Constant  Value=0
  Constant3 : Constant  Value=0
  Demux : Demux
  Demux1 : Demux
  Divide : Product  Inputs=*/
  Integrator : Integrator  WrapState=on
  Interpreted MATLAB Function : MATLABFcn  MATLABFcn=quat2rotm(u)  Output1D=off
  MATLAB Function : MATLAB Function  TreatAsAtomicUnit=on
  Mux : Mux
  Mux1 : Mux
  Subsystem : Subsystem
      mask Display: image('$imagefile'); % Use "Edit Image" on toolstrip to change.
  Sum : Sum  Inputs=++|
  Switch : Switch  Criteria=u2 ~= 0  SaturateOnIntegerOverflow=off  InputSameDT=off
  Terminator{,1..7} (8 alike) : Terminator
  Vector Concatenate : Concatenate
  mixer : Subsystem
  plant : Subsystem
      settings: PortSchema="{\"entries\":[{\"content\":{\"sides\":[{\"content\":{\"connectorIds\":[\"In1\"]},\"type\":\"ConnectorPlacement.EquallySpacedRectSide\",\"uuid\":\"6e9c785b-7a58-4a83-84e6-bbea81e0823c\"},{\"content\":{\"connectorIds\":[\"Out1\",\"Out2\",\"Out3\",\"Out4\",\"Out5\",\"Out6\",\"Out7\",\"Out8\"],\"side\":\"RIGHT\"},\"type\":\"ConnectorPlacement.EquallySpacedRectSide\",\"uuid\":\"b008e1e2-aa95-4897-b360-2fe655e93601\"},{\"content\":{\"connectorIds\":[],\"side\":\"TOP\"},\"type\":\"ConnectorPlacement.EquallySpacedRectSide\",\"uuid\":\"363cdb01-a5e5-4a3c-bce9-213e2ffac7b5\"},{\"content\":{\"connectorIds\":[\"RConn1\",\"RConn2\"],\"side\":\"BOTTOM\"},\"type\":\"ConnectorPlacement.EquallySpacedRectSide\",\"uuid\":\"8e0d8754-e9ec-4386-98a0-719833eb7e87\"}]},\"type\":\"ConnectorPlacement.EquallySpacedConnector\",\"uuid\":\"eb300e37-0abf-4331-8664-ac63688da223\"}],\"packageUris\":[\"http://schema.mathworks.com/mf0/Connector/R2020b\"],\"version\":\"1.0\"}"
      mask Display: image('$imagefile'); % Use "Edit Image" on toolstrip to change.
  position controller : Subsystem
      mask Display: image('$imagefile'); % Use "Edit Image" on toolstrip to change.
  quat 2 euler (ROS) : MATLAB Function  TreatAsAtomicUnit=on
  quat 2 euler (UE) : MATLAB Function  TreatAsAtomicUnit=on
  base : PMIOPort  Side=Right
  collision : PMIOPort  Port=2  Side=Right
  position : Outport
  position_ue : Outport  Port=2
  attitude_ue : Outport  Port=3
  wires:
  plant/4(quaternion) -> quat 2 euler (ROS)/1(q), Terminator6/1, Interpreted MATLAB Function/1
  plant/6(angular_acceleration [rad/s^2]) -> Terminator/1
  plant/3(acceleration [m/s^2]) -> Terminator1/1
  Interpreted MATLAB Function/1 -> MATLAB Function/1(u), Subsystem/5(rotation_matrix)
  plant/5(angular_velocity [m/s]) -> Terminator7/1, Subsystem/6(angular_velocity [rad/s])
  quat 2 euler (UE)/1(attitude) -> attitude_ue/1
  plant/8(quaternion_ue) -> quat 2 euler (UE)/1(q)
  plant/7(position_ue [m]) -> position_ue/1
  plant/2(velocity [m/s]) -> Terminator5/1, position controller/2(velocity [m/s])
  plant/1(position [m]) -> position controller/1(position [m]), position/1
  Constant2/1 -> Subsystem/4(setpoint_yaw_rate [rad/s])
  setpoint_acceleration/1 -> position controller/5(setpoint_acceleration [m/s^2])
  setpoint_velocity/1 -> position controller/4(setpoint_velocity [m/s])
  setpoint_position/1 -> position controller/3(setpoint_position [m])
  Constant3/1 -> Mux/4, position controller/6(yaw [rad])
  quat 2 euler (ROS)/1(roll_rad) -> Terminator2/1
  quat 2 euler (ROS)/2(pitch_rad) -> Terminator3/1
  quat 2 euler (ROS)/3(yaw_rad) -> Terminator4/1
  position controller/1(thrust [N]) -> Mux/1
  position controller/2(roll [rad]) -> Mux/2
  position controller/3(pitch [rad]) -> Mux/3
  Demux/2 -> Subsystem/1(setpoint_roll [rad])
  Demux/3 -> Subsystem/2(setpoint_pitch [rad])
  Demux/4 -> Subsystem/3(setpoint_yaw [rad])
  Switch/1 -> Demux/1
  Mux/1 -> Switch/3
  joystick_on/1 -> Switch/2
  joystick/1 -> Demux1/1
  Demux1/2 -> Mux1/2
  Demux1/3 -> Mux1/3
  Mux1/1 -> Switch/1
  Demux1/4 -> Integrator/1
  Integrator/1 -> Mux1/4
  Sum/1 -> Mux1/1
  Constant/1 -> Sum/1
  Demux1/1 -> Sum/2
  Demux/1 -> Divide/1
  Divide/1 -> Vector Concatenate/1
  Subsystem/1(torques [N*m]) -> Vector Concatenate/2
  MATLAB Function/1(y) -> Divide/2
  Vector Concatenate/1 -> mixer/1(In1)
  mixer/1(Out1) -> plant/1(motor_velocities [rad/s])
  connections:
  plant/RConn1 -- base/RConn1
  collision/RConn1 -- plant/RConn2

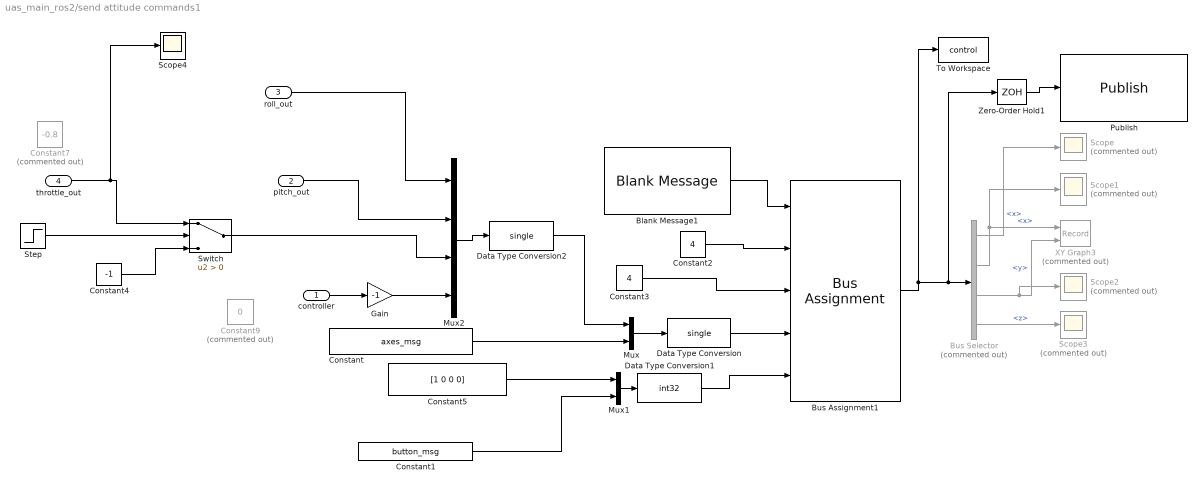
== system uas_main_ros2/send attitude commands1 ==
  controller : Inport
  pitch_out : Inport  Port=2
  roll_out : Inport  Port=3
  throttle_out : Inport  Port=4
  Blank Message1 : ros2lib/Blank Message  messageClass=Message  entityType=sensor_msgs/Joy  messageType=sensor_msgs/Joy  SampleTime=inf
  Bus Assignment1 : BusAssignment  AssignedSignals=axes_SL_Info.CurrentLength,buttons_SL_Info.CurrentLength,axes,buttons
  Bus Selector : BusSelector  Commented=on  OutputSignals=linear.x,angular.x,angular.y,angular.z
  Constant : Constant  Value=axes_msg  OutDataTypeStr=single
  Constant1 : Constant  Value=button_msg  OutDataTypeStr=int32  LockScale=on
  Constant2 : Constant  Value=4  OutDataTypeStr=uint32
  Constant3 : Constant  Value=4  OutDataTypeStr=uint32
  Constant4 : Constant  Value=-1
  Constant5 : Constant  Value=[1 0 0 0]  OutDataTypeStr=int32
  Constant7 : Constant  Commented=on  Value=-0.8  OutDataTypeStr=double
  Constant9 : Constant  Commented=on  Value=0  OutDataTypeStr=double
  Data Type Conversion : DataTypeConversion  OutDataTypeStr=single  SaturateOnIntegerOverflow=off  RndMeth=Floor
  Data Type Conversion1 : DataTypeConversion  OutDataTypeStr=int32  SaturateOnIntegerOverflow=off  RndMeth=Floor
  Data Type Conversion2 : DataTypeConversion  OutDataTypeStr=single  SaturateOnIntegerOverflow=off  RndMeth=Floor
  Gain : Gain  Gain=-1
  Mux : Mux  Inputs=2
  Mux1 : Mux  Inputs=2
  Mux2 : Mux
  Publish : ros2lib/Publish  topicSource=Specify your own  topic=/joy  messageType=sensor_msgs/Joy  QOSHistory=Keep last  QOSDepth=1  QOSReliability=Reliable  QOSDurability=Volatile  QOSDeadline=Inf  QOSLifespan=Inf  QOSLiveliness=Automatic  QOSLeaseDuration=Inf  QOSAvoidROSNamespaceConventions=off
  Scope{,1..3} (4 alike) : Scope  Commented=on
      Scope settings: ActiveDisplayYMinimum=500  ActiveDisplayYMaximum=2500  DataLoggingVariableName=ScopeData4
      Scope1 settings: ActiveDisplayYMinimum=500  ActiveDisplayYMaximum=2500  DataLoggingVariableName=ScopeData5
      Scope2 settings: ActiveDisplayYMinimum=-1  ActiveDisplayYMaximum=1  DataLoggingVariableName=ScopeData6
      Scope3 settings: ActiveDisplayYMinimum=-1  ActiveDisplayYMaximum=1  DataLoggingVariableName=ScopeData7
  Scope4 : Scope
      settings: ActiveDisplayYMinimum=-0.59568705733108451  ActiveDisplayYMaximum=0.5179877790240347  DataLoggingVariableName=ScopeData14
  Step : Step  Time=0.5  SampleTime=sample_time
  Switch : Switch  Criteria=u2 > Threshold  SaturateOnIntegerOverflow=off  InputSameDT=off
  To Workspace : ToWorkspace  VariableName=control  SaveFormat=Timeseries  SampleTime=-1
  XY Graph3 : Record  Commented=on  NumPorts=2.0  FileSettingsInternal="{\"entries\":[{\"content\":{\"excelSettings\":{\"content\":{},\"type\":\"Streamout.ExcelSettings\"},\"parquetSettings\":{\"content\":{},\"type\":\"Streamout.ParquetSettings\"}},\"type\":\"Streamout.FileSettingStorage\",\"uuid\":\"\"}],\"packageUris\":[\"http:\\/\\/schema.mathworks.com\\/mf0\\/streamout_blocks\\/R2020a\"],\"version\":\"1.0\"}"  FrameSettings=[0, 0]  Layout=[1 1]  SignalsInternal="{\"entries\":[{\"content\":{\"signals\":[{\"content\":{\"blockPath\":[],\"dimensions\":[1],\"domain\":\"\",\"lineColor\":\"#0072bd\",\"lineWidth\":2,\"port\":1,\"signalID\":1,\"signalName\":\"<x>\"},\"type\":\"RecordBlkView.Signal\",\"uuid\":\"\"},{\"content\":{\"blockPath\":[],\"dimensions\":[1],\"domain\":\"\",\"lineColor\":\"#d95319\",\"lineWidth\":2,\"port\":2,\"signalID\":2,\"signalName\":\"<y>\"},\"type\":\"RecordBlkView.Signal\",\"uuid\":\"\"}]},\"type\":\"RecordBlkView.InputSignals\",\"uuid\":\"\"}],\"packageUris\":[\"http:\\/\\/schema.mathworks.com\\/mf0\\/streamout_blocks\\/R2020a\"],\"version\":\"1.0\"}"  VisualizationBindings="{\"xyplotplugin\":{\"info\":[{\"series\":[],\"subplotID\":1}]}}"  CompatibilityTag=XY
  Zero-Order Hold1 : ZeroOrderHold  SampleTime=sample_time
  wires:
  Bus Selector/4 -> Scope3/1  "<z>"
  Bus Selector/2 -> XY Graph3/1, Scope1/1  "<x>"
  Bus Selector/3 -> XY Graph3/2, Scope2/1  "<y>"
  Zero-Order Hold1/1 -> Publish/1
  Bus Assignment1/1 -> Bus Selector/1, Zero-Order Hold1/1, To Workspace/1
  Bus Selector/1 -> Scope/1  "<x>"
  Blank Message1/1 -> Bus Assignment1/1
  Constant2/1 -> Bus Assignment1/2
  Constant3/1 -> Bus Assignment1/3
  Constant/1 -> Mux/2
  Mux2/1 -> Data Type Conversion2/1
  Constant1/1 -> Mux1/2
  Constant5/1 -> Mux1/1
  Switch/1 -> Mux2/3
  controller/1 -> Gain/1
  Data Type Conversion/1 -> Bus Assignment1/4
  Data Type Conversion1/1 -> Bus Assignment1/5
  throttle_out/1 -> Scope4/1, Switch/1
  Constant4/1 -> Switch/3
  Step/1 -> Switch/2
  Data Type Conversion2/1 -> Mux/1
  Mux/1 -> Data Type Conversion/1
  Mux1/1 -> Data Type Conversion1/1
  Gain/1 -> Mux2/4
  pitch_out/1 -> Mux2/2
  roll_out/1 -> Mux2/1

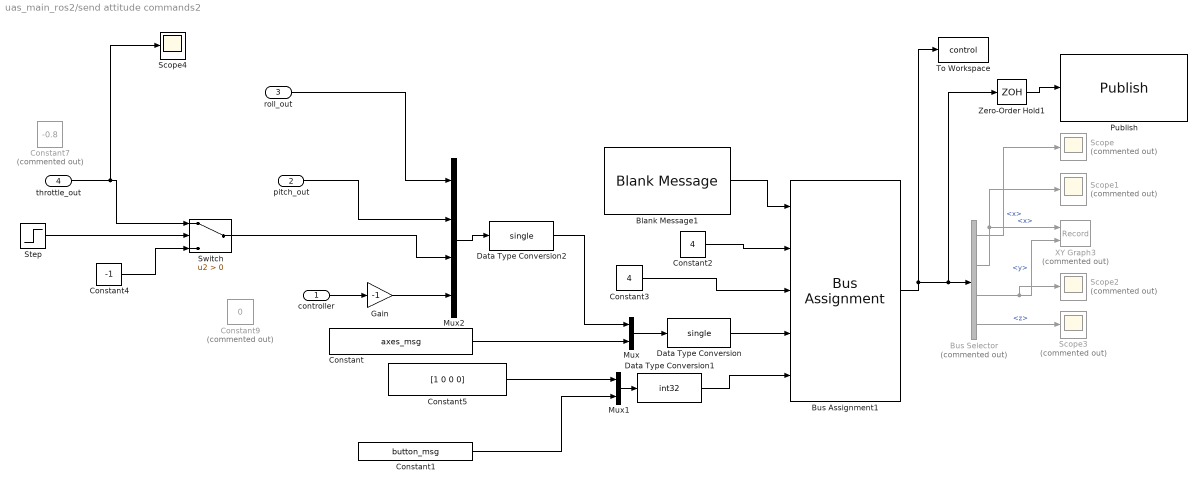
== system uas_main_ros2/send attitude commands2 ==
  controller : Inport
  pitch_out : Inport  Port=2
  roll_out : Inport  Port=3
  throttle_out : Inport  Port=4
  Blank Message1 : ros2lib/Blank Message  messageClass=Message  entityType=sensor_msgs/Joy  messageType=sensor_msgs/Joy  SampleTime=inf
  Bus Assignment1 : BusAssignment  AssignedSignals=axes_SL_Info.CurrentLength,buttons_SL_Info.CurrentLength,axes,buttons
  Bus Selector : BusSelector  Commented=on  OutputSignals=linear.x,angular.x,angular.y,angular.z
  Constant : Constant  Value=axes_msg  OutDataTypeStr=single
  Constant1 : Constant  Value=button_msg  OutDataTypeStr=int32  LockScale=on
  Constant2 : Constant  Value=4  OutDataTypeStr=uint32
  Constant3 : Constant  Value=4  OutDataTypeStr=uint32
  Constant4 : Constant  Value=-1
  Constant5 : Constant  Value=[1 0 0 0]  OutDataTypeStr=int32
  Constant7 : Constant  Commented=on  Value=-0.8  OutDataTypeStr=double
  Constant9 : Constant  Commented=on  Value=0  OutDataTypeStr=double
  Data Type Conversion : DataTypeConversion  OutDataTypeStr=single  SaturateOnIntegerOverflow=off  RndMeth=Floor
  Data Type Conversion1 : DataTypeConversion  OutDataTypeStr=int32  SaturateOnIntegerOverflow=off  RndMeth=Floor
  Data Type Conversion2 : DataTypeConversion  OutDataTypeStr=single  SaturateOnIntegerOverflow=off  RndMeth=Floor
  Gain : Gain  Gain=-1
  Mux : Mux  Inputs=2
  Mux1 : Mux  Inputs=2
  Mux2 : Mux
  Publish : ros2lib/Publish  topicSource=Specify your own  topic=/joy  messageType=sensor_msgs/Joy  QOSHistory=Keep last  QOSDepth=1  QOSReliability=Reliable  QOSDurability=Volatile  QOSDeadline=Inf  QOSLifespan=Inf  QOSLiveliness=Automatic  QOSLeaseDuration=Inf  QOSAvoidROSNamespaceConventions=off
  Scope{,1..3} (4 alike) : Scope  Commented=on
      Scope settings: ActiveDisplayYMinimum=500  ActiveDisplayYMaximum=2500  DataLoggingVariableName=ScopeData4
      Scope1 settings: ActiveDisplayYMinimum=500  ActiveDisplayYMaximum=2500  DataLoggingVariableName=ScopeData5
      Scope2 settings: ActiveDisplayYMinimum=-1  ActiveDisplayYMaximum=1  DataLoggingVariableName=ScopeData6
      Scope3 settings: ActiveDisplayYMinimum=-1  ActiveDisplayYMaximum=1  DataLoggingVariableName=ScopeData7
  Scope4 : Scope
      settings: ActiveDisplayYMinimum=0.21428938400516886  ActiveDisplayYMaximum=0.96098064847348419  DataLoggingVariableName=ScopeData14
  Step : Step  Time=0.5  SampleTime=sample_time
  Switch : Switch  Criteria=u2 > Threshold  SaturateOnIntegerOverflow=off  InputSameDT=off
  To Workspace : ToWorkspace  VariableName=control  SaveFormat=Timeseries  SampleTime=-1
  XY Graph3 : Record  Commented=on  NumPorts=2.0  FileSettingsInternal="{\"entries\":[{\"content\":{\"excelSettings\":{\"content\":{},\"type\":\"Streamout.ExcelSettings\"},\"parquetSettings\":{\"content\":{},\"type\":\"Streamout.ParquetSettings\"}},\"type\":\"Streamout.FileSettingStorage\",\"uuid\":\"\"}],\"packageUris\":[\"http:\\/\\/schema.mathworks.com\\/mf0\\/streamout_blocks\\/R2020a\"],\"version\":\"1.0\"}"  FrameSettings=[0, 0]  Layout=[1 1]  SignalsInternal="{\"entries\":[{\"content\":{\"signals\":[{\"content\":{\"blockPath\":[],\"dimensions\":[1],\"domain\":\"\",\"lineColor\":\"#0072bd\",\"lineWidth\":2,\"port\":1,\"signalID\":1,\"signalName\":\"<x>\"},\"type\":\"RecordBlkView.Signal\",\"uuid\":\"\"},{\"content\":{\"blockPath\":[],\"dimensions\":[1],\"domain\":\"\",\"lineColor\":\"#d95319\",\"lineWidth\":2,\"port\":2,\"signalID\":2,\"signalName\":\"<y>\"},\"type\":\"RecordBlkView.Signal\",\"uuid\":\"\"}]},\"type\":\"RecordBlkView.InputSignals\",\"uuid\":\"\"}],\"packageUris\":[\"http:\\/\\/schema.mathworks.com\\/mf0\\/streamout_blocks\\/R2020a\"],\"version\":\"1.0\"}"  VisualizationBindings="{\"xyplotplugin\":{\"info\":[{\"series\":[],\"subplotID\":1}]}}"  CompatibilityTag=XY
  Zero-Order Hold1 : ZeroOrderHold  SampleTime=sample_time
  wires:
  Bus Selector/4 -> Scope3/1  "<z>"
  Bus Selector/2 -> XY Graph3/1, Scope1/1  "<x>"
  Bus Selector/3 -> XY Graph3/2, Scope2/1  "<y>"
  Zero-Order Hold1/1 -> Publish/1
  Bus Assignment1/1 -> Bus Selector/1, Zero-Order Hold1/1, To Workspace/1
  Bus Selector/1 -> Scope/1  "<x>"
  Blank Message1/1 -> Bus Assignment1/1
  Constant2/1 -> Bus Assignment1/2
  Constant3/1 -> Bus Assignment1/3
  Constant/1 -> Mux/2
  Mux2/1 -> Data Type Conversion2/1
  Constant1/1 -> Mux1/2
  Constant5/1 -> Mux1/1
  Switch/1 -> Mux2/3
  controller/1 -> Gain/1
  Data Type Conversion/1 -> Bus Assignment1/4
  Data Type Conversion1/1 -> Bus Assignment1/5
  throttle_out/1 -> Scope4/1, Switch/1
  Constant4/1 -> Switch/3
  Step/1 -> Switch/2
  Data Type Conversion2/1 -> Mux/1
  Mux/1 -> Data Type Conversion/1
  Mux1/1 -> Data Type Conversion1/1
  Gain/1 -> Mux2/4
  pitch_out/1 -> Mux2/2
  roll_out/1 -> Mux2/1
